simulink model "basalMode2023a"  (R2023a)
settings: Solver=VariableStepAuto  StartTime=0.0  StopTime=10.0  RelTol=1e-3
settings Model: Creator=anson  LastModifiedBy=anson

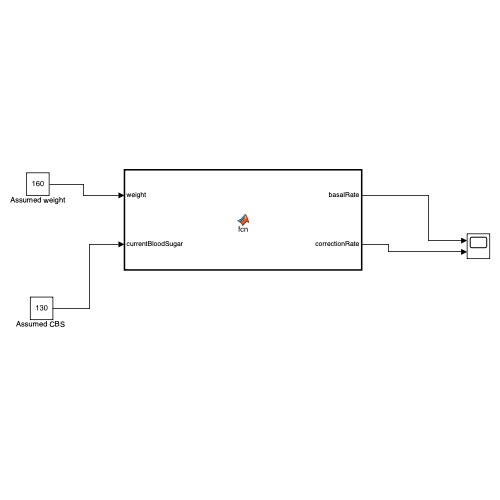
[thumbnail: Simulink's stored preview of the top-level diagram]
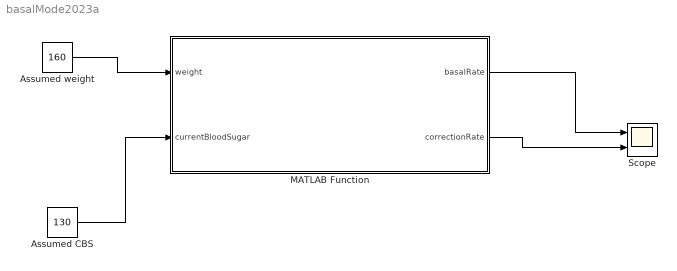
== system basalMode2023a ==
  "Assumed CBS " : Constant  Value=130
  Assumed weight : Constant  Value=160
  MATLAB Function : MATLAB Function  TreatAsAtomicUnit=on
  Scope : Scope  NumInputPorts=2
  wires:
  Assumed weight/1 -> MATLAB Function/1(weight)
  "Assumed CBS "/1 -> MATLAB Function/2(currentBloodSugar)
  MATLAB Function/1(basalRate) -> Scope/1
  MATLAB Function/2(correctionRate) -> Scope/2

== matlab function basalMode2023a/MATLAB Function ==
  data: weight input; basalRate output; currentBloodSugar input; correctionRate output
function [basalRate, correctionRate]= fcn(weight, currentBloodSugar)

    % Constants
    TARGET_BLOOD_SUGAR = 100; % Target blood sugar level in mg/dl
    CORRECTION_FACTOR_CONSTANT = 1800; % Constant for correction factor calculation

    % Total Daily Insulin Dose (TDI)
    totalDailyInsulin = weight / 4;

    % Basal/background Insulin Dose
    basalDose = 0.5 * totalDailyInsulin; % 50% of TDI

    % Basal Insulin Delivery Rate per min
    basalRate = basalDose / 24 / 60; % Delivery rate per minute

    % Correction Factor
    correctionFactor = CORRECTION_FACTOR_CONSTANT / totalDailyInsulin;

    % Correction Dose Calculation
    if currentBloodSugar > 120 % High blood sugar state
        correctionDose = (currentBloodSugar - TARGET_BLOOD_SUGAR) / correctionFactor;
    elseif currentBloodSugar < 80 % Low blood sugar state
        basalRate = 0; % Suspend basal insulin delivery
        correctionDose = 0;
    else
        correctionDose = 0; % Normal blood sugar state
    end
    
    correctionRate = correctionDose % Correction Rate per minute
    
end
